simulink model "simWilczkiOwieczki"  (R2012b)
settings: Solver=ode45  StartTime=0.0  StopTime=10  RelTol=1e-3
values from neighbouring files (symbols this model uses):
  narodzinyOwiec = 3    [zad2_3.m]
  narodzinyWilkow = 1.1    [zad2_3.m]
  owce = 7    [zad2_3.m]
  podzialka = 0.00003    (= 3e-05)    [zad2_3.m]
  wilki = 7    [zad2_3.m]
  zgonyOwiec = 1    [zad2_3.m]
  zgonyWilkow = 0.7    [zad2_3.m]
settings Model: Creator=Jonatan  LastModifiedBy=Elejdor
settings DataIOCC: SignalLoggingSaveFormat=ModelDataLogs
settings OptimizationCC: ExpressionDepthLimit=128
settings DebuggingCC: MultiTaskDSMMsg=warning  MultiTaskCondExecSysMsg=none  StateNameClashWarn=none  StrictBusMsg=None
settings RTWCC: IncludeERTFirstTime=on
settings CodeAppCC: CustomSymbolStrType=$N$R$M_T  InternalIdentifier=Shortened

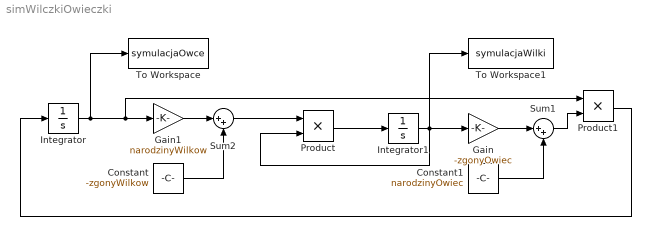
== system simWilczkiOwieczki ==
  Constant : Constant  Value=-zgonyWilkow  SampleTime=podzialka
  Constant1 : Constant  Value=narodzinyOwiec  SampleTime=podzialka
  Gain : Gain  Gain=-zgonyOwiec  SampleTime=podzialka
  Gain1 : Gain  Gain=narodzinyWilkow  SampleTime=podzialka
  Integrator : Integrator  InitialCondition=owce  LowerSaturationLimit=0
  Integrator1 : Integrator  InitialCondition=wilki  LowerSaturationLimit=0
  Product : Product  SampleTime=podzialka
  Product1 : Product  SampleTime=podzialka
  Sum1 : Sum  Inputs=|++  SampleTime=podzialka
  Sum2 : Sum  Inputs=|++  SampleTime=podzialka
  To Workspace : ToWorkspace  VariableName=symulacjaOwce  SampleTime=podzialka
  To Workspace1 : ToWorkspace  VariableName=symulacjaWilki  SampleTime=podzialka
  wires:
  Integrator1/1 -> Gain/1, Product/2, To Workspace1/1
  Product1/1 -> Integrator/1
  Sum2/1 -> Product/1
  Sum1/1 -> Product1/2
  Constant/1 -> Sum2/2
  Constant1/1 -> Sum1/2
  Gain/1 -> Sum1/1
  Gain1/1 -> Sum2/1
  Product/1 -> Integrator1/1
  Integrator/1 -> To Workspace/1, Product1/1, Gain1/1
